simulink model "ComauSMARTS2_CL"  (R2018b)
settings: Solver=ode1  StartTime=0.0  StopTime=tf  FixedStep=T  RelTol=1e-3
values from neighbouring files (symbols this model uses):
  dotq0_ = [0 0 0]    [main.m]
  Kd1 = 1e3    (= 1000)    [main.m]
  Kd2 = 5e2    (= 500)    [main.m]
  Kd3 = 200    [main.m]
  Ki1 = 1e1    (= 10)    [main.m]
  Ki2 = 5e1    (= 50)    [main.m]
  Ki3 = 2    [main.m]
  Kp1 = 1e4    (= 10000)    [main.m]
  Kp2 = 5e3    (= 5000)    [main.m]
  Kp3 = 4e3    (= 4000)    [main.m]
  l1 = 0.65    [main.m]
  l2 = 0.6576    [main.m]
  q0_ = [1.4 0.9 1.1]    [main.m]
  qd_ = [pi/2 pi/4 pi/3]    [main.m]
undefined symbols (not defined in the file or in its folder): gamma
libraries: dspmtrx3 x4, dspinverses x1
settings Model: SimulationMode=accelerator  Creator=gpinc  LastModifiedBy=corrado
settings SFSimCC: SimUseLocalCustomCode=off
settings RTWCC: RTWUseLocalCustomCode=off
settings CodeAppCC: StateflowObjectComments=on

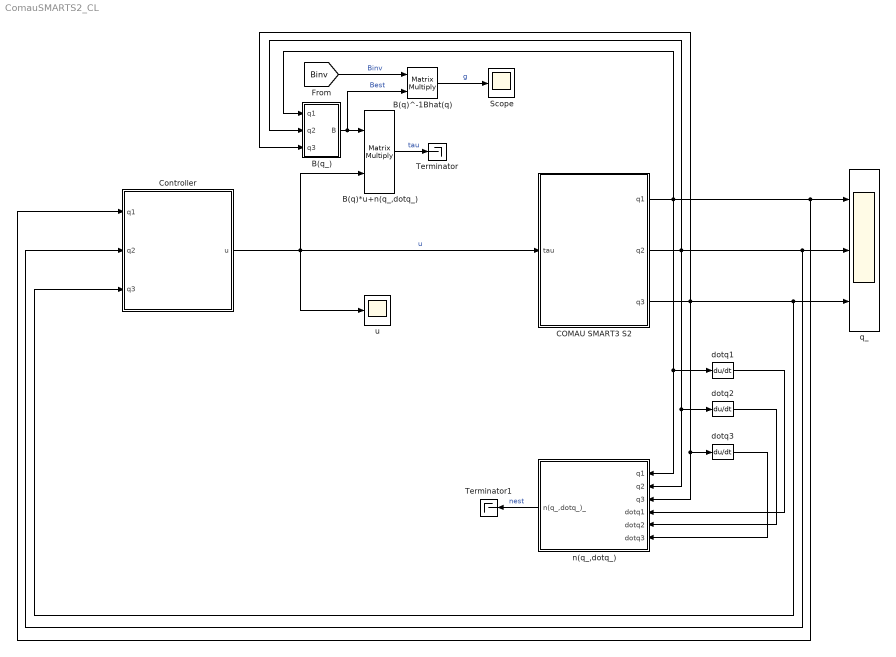
== system ComauSMARTS2_CL ==
  B(q)*u+n(q_,dotq_) : Product  Multiplication=Matrix(*)  RndMeth=Zero
  B(q)^-1Bhat(q) : Product  Multiplication=Matrix(*)  RndMeth=Zero
  B(q_) : Subsystem
  COMAU SMART3 S2 : Subsystem
      mask Display: image(imread('SMARTS2.jpeg'))
  Controller : Subsystem
  Scope : Scope
  Terminator : Terminator
  Terminator1 : Terminator
  dotq1 : Derivative
  dotq2 : Derivative
  dotq3 : Derivative
  n(q_,dotq_) : Subsystem
  q_ : Scope  NumInputPorts=3
  u : Scope
  wires:
  dotq1/1 -> n(q_,dotq_)/4(dotq1)
  B(q_)/1(B) -> B(q)^-1Bhat(q)/2, B(q)*u+n(q_,dotq_)/1  "Best"
  Controller/1(u) -> COMAU SMART3 S2/1(tau), u/1, B(q)*u+n(q_,dotq_)/2  "u"
  COMAU SMART3 S2/2(q2) -> dotq2/1, n(q_,dotq_)/2(q2), B(q_)/2(q2), q_/2, Controller/2(q2)
  dotq3/1 -> n(q_,dotq_)/6(dotq3)
  COMAU SMART3 S2/3(q3) -> dotq3/1, n(q_,dotq_)/3(q3), B(q_)/3(q3), q_/3, Controller/3(q3)
  COMAU SMART3 S2/1(q1) -> dotq1/1, n(q_,dotq_)/1(q1), B(q_)/1(q1), q_/1, Controller/1(q1)
  dotq2/1 -> n(q_,dotq_)/5(dotq2)
  [Binv] -> B(q)^-1Bhat(q)/1  "Binv"
  B(q)^-1Bhat(q)/1 -> Scope/1  "g"
  B(q)*u+n(q_,dotq_)/1 -> Terminator/1  "tau"
  n(q_,dotq_)/1(n(q_,dotq_)_) -> Terminator1/1  "nest"

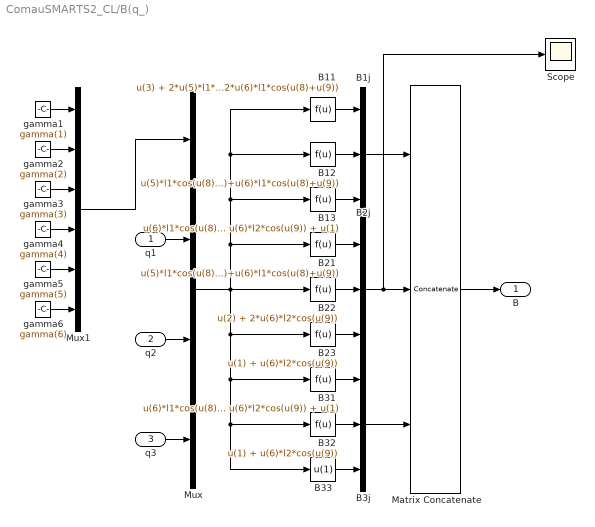
== system ComauSMARTS2_CL/B(q_) ==
  q1 : Inport
  q2 : Inport  Port=2
  q3 : Inport  Port=3
  B11 : Fcn  Expr=u(3) + 2*u(5)*l1*cos(u(8)) + 2*u(6)*l2*cos(u(9)) + 2*u(6)*l1*cos(u(8)+u(9))
  B12 : Fcn  Expr=u(5)*l1*cos(u(8))+u(2)+2*u(6)*l2*cos(u(9))+u(6)*l1*cos(u(8)+u(9))
  B13 : Fcn  Expr=u(6)*l1*cos(u(8)+u(9)) + u(6)*l2*cos(u(9)) + u(1)
  B1j : Concatenate  NumInputs=3
  B21 : Fcn  Expr=u(5)*l1*cos(u(8))+u(2)+2*u(6)*l2*cos(u(9))+u(6)*l1*cos(u(8)+u(9))
  B22 : Fcn  Expr=u(2) + 2*u(6)*l2*cos(u(9))
  B23 : Fcn  Expr=u(1) + u(6)*l2*cos(u(9))
  B2j : Concatenate  NumInputs=3
  B31 : Fcn  Expr=u(6)*l1*cos(u(8)+u(9)) + u(6)*l2*cos(u(9)) + u(1)
  B32 : Fcn  Expr=u(1) + u(6)*l2*cos(u(9))
  B33 : Fcn  Expr=u(1)
  B3j : Concatenate  NumInputs=3
  Matrix Concatenate : Concatenate  NumInputs=3  Mode=Multidimensional array  ConcatenateDimension=2
  Mux : Mux
  Mux1 : Mux  Inputs=6
  Scope : Scope
  gamma1 : Constant  Value=gamma(1)
  gamma2 : Constant  Value=gamma(2)
  gamma3 : Constant  Value=gamma(3)
  gamma4 : Constant  Value=gamma(4)
  gamma5 : Constant  Value=gamma(5)
  gamma6 : Constant  Value=gamma(6)
  B : Outport
  wires:
  B11/1 -> B1j/1
  B33/1 -> B3j/3
  B12/1 -> B1j/2
  B13/1 -> B1j/3
  B22/1 -> B2j/2
  B23/1 -> B2j/3
  B21/1 -> B2j/1
  B31/1 -> B3j/1
  B32/1 -> B3j/2
  Mux/1 -> B22/1, B21/1, B11/1, B12/1, B13/1, B23/1, B31/1, B32/1, B33/1
  Matrix Concatenate/1 -> B/1
  B3j/1 -> Matrix Concatenate/3
  B2j/1 -> Scope/1, Matrix Concatenate/2
  B1j/1 -> Matrix Concatenate/1
  q3/1 -> Mux/4
  q2/1 -> Mux/3
  q1/1 -> Mux/2
  Mux1/1 -> Mux/1
  gamma6/1 -> Mux1/6
  gamma5/1 -> Mux1/5
  gamma4/1 -> Mux1/4
  gamma3/1 -> Mux1/3
  gamma2/1 -> Mux1/2
  gamma1/1 -> Mux1/1

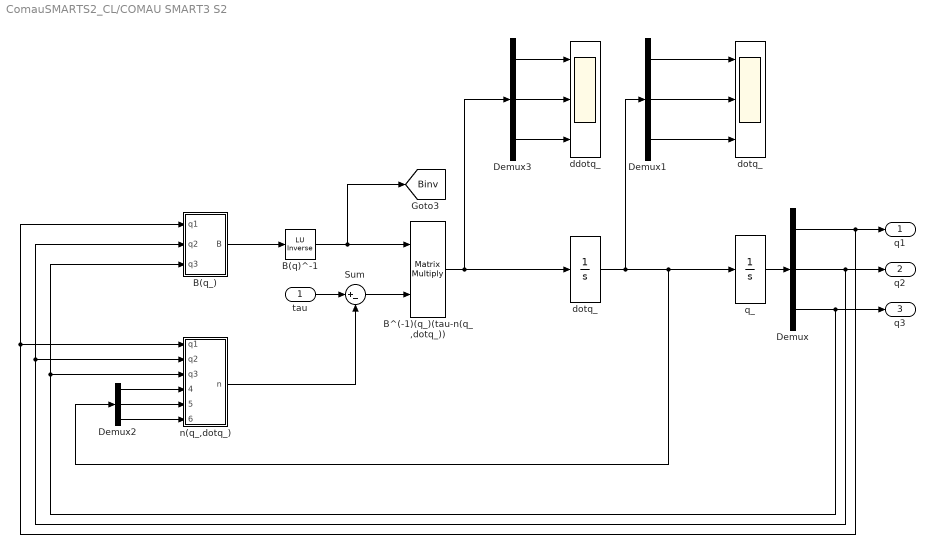
== system ComauSMARTS2_CL/COMAU SMART3 S2 ==
  tau : Inport
  " B(q)^-1" : dspinverses/ LU Inverse
      settings: SourceProductName=DSP System Toolbox
  B(q_) : Subsystem
  B^(-1)(q_)(tau-n(q_,dotq_)) : Product  Multiplication=Matrix(*)  RndMeth=Zero
  Demux{,1..3} (4 alike) : Demux  Outputs=3
  Sum : Sum  Inputs=|+-
  ddotq_ : Scope  NumInputPorts=3
  dotq_ : Integrator  InitialCondition=dotq0_
  "dotq_ " : Scope  NumInputPorts=3
  n(q_,dotq_) : Subsystem
  q_ : Integrator  InitialCondition=q0_
  q1 : Outport
  q2 : Outport  Port=2
  q3 : Outport  Port=3
  tag scope: Binv=global
  wires:
  dotq_/1 -> q_/1, Demux2/1, Demux1/1
  q_/1 -> Demux/1
  B(q_)/1(B) -> " B(q)^-1"/1
  Demux/3 -> q3/1, B(q_)/3(q3), n(q_,dotq_)/3(q3)
  Demux/2 -> q2/1, B(q_)/2(q2), n(q_,dotq_)/2(q2)
  Demux/1 -> q1/1, B(q_)/1(q1), n(q_,dotq_)/1(q1)
  Demux1/3 -> "dotq_ "/3
  Demux1/2 -> "dotq_ "/2
  Demux1/1 -> "dotq_ "/1
  n(q_,dotq_)/1(n) -> Sum/2
  " B(q)^-1"/1 -> [Binv], B^(-1)(q_)(tau-n(q_,dotq_))/1
  Sum/1 -> B^(-1)(q_)(tau-n(q_,dotq_))/2
  Demux3/3 -> ddotq_/3
  Demux3/2 -> ddotq_/2
  tau/1 -> Sum/1
  Demux2/1 -> n(q_,dotq_)/4(dotq1)
  Demux3/1 -> ddotq_/1
  B^(-1)(q_)(tau-n(q_,dotq_))/1 -> Demux3/1, dotq_/1
  Demux2/2 -> n(q_,dotq_)/5(dotq2)
  Demux2/3 -> n(q_,dotq_)/6(dotq3)

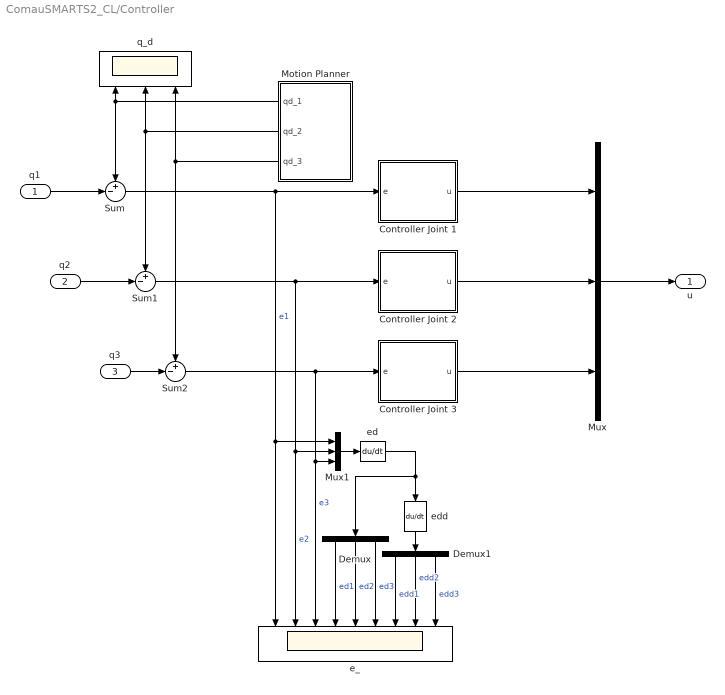
== system ComauSMARTS2_CL/Controller ==
  q1 : Inport
  q2 : Inport  Port=2
  q3 : Inport  Port=3
  Controller Joint 1 : Subsystem
  Controller Joint 2 : Subsystem
  Controller Joint 3 : Subsystem
  Demux : Demux  Outputs=3
  Demux1 : Demux  Outputs=3
  Motion Planner : Subsystem
  Mux : Mux  Inputs=3
  Mux1 : Mux  Inputs=3
  Sum : Sum  Inputs=+-|
  Sum1 : Sum  Inputs=+-|
  Sum2 : Sum  Inputs=+-|
  e_ : Scope  NumInputPorts=9
  ed : Derivative
  edd : Derivative
  q_d : Scope  NumInputPorts=3
  u : Outport
  wires:
  q1/1 -> Sum/2
  q2/1 -> Sum1/2
  q3/1 -> Sum2/2
  Sum/1 -> e_/1, Mux1/1, Controller Joint 1/1(e)  "e1"
  Sum1/1 -> e_/2, Mux1/2, Controller Joint 2/1(e)  "e2"
  Controller Joint 3/1(u) -> Mux/3
  Sum2/1 -> Controller Joint 3/1(e), e_/3, Mux1/3  "e3"
  Mux1/1 -> ed/1
  Demux/1 -> e_/4  "ed1"
  Demux/2 -> e_/5  "ed2"
  Demux/3 -> e_/6  "ed3"
  Demux1/1 -> e_/7  "edd1"
  Demux1/2 -> e_/8  "edd2"
  Demux1/3 -> e_/9  "edd3"
  Controller Joint 2/1(u) -> Mux/2
  Controller Joint 1/1(u) -> Mux/1
  edd/1 -> Demux1/1
  ed/1 -> edd/1, Demux/1
  Mux/1 -> u/1
  Motion Planner/3(qd_3) -> q_d/3, Sum2/1
  Motion Planner/2(qd_2) -> Sum1/1, q_d/2
  Motion Planner/1(qd_1) -> q_d/1, Sum/1

== system ComauSMARTS2_CL/n(q_,dotq_) ==
  q1 : Inport
  q2 : Inport  Port=2
  q3 : Inport  Port=3
  dotq1 : Inport  Port=4
  dotq2 : Inport  Port=5
  dotq3 : Inport  Port=6
  n(q_,dotq_) : Subsystem
  n(q_,dotq_)_ : Outport
  wires:
  q1/1 -> n(q_,dotq_)/1(q1)
  q2/1 -> n(q_,dotq_)/2(q2)
  q3/1 -> n(q_,dotq_)/3(q3)
  n(q_,dotq_)/1(n) -> n(q_,dotq_)_/1
  dotq1/1 -> n(q_,dotq_)/4(dotq1)
  dotq2/1 -> n(q_,dotq_)/5(dotq2)
  dotq3/1 -> n(q_,dotq_)/6(dotq3)

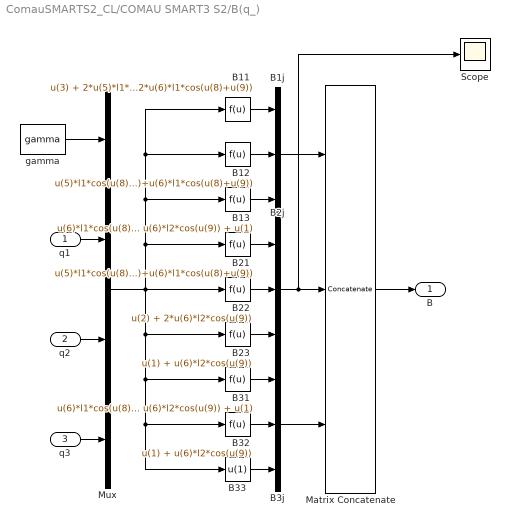
== system ComauSMARTS2_CL/COMAU SMART3 S2/B(q_) ==
  q1 : Inport
  q2 : Inport  Port=2
  q3 : Inport  Port=3
  B11 : Fcn  Expr=u(3) + 2*u(5)*l1*cos(u(8)) + 2*u(6)*l2*cos(u(9)) + 2*u(6)*l1*cos(u(8)+u(9))
  B12 : Fcn  Expr=u(5)*l1*cos(u(8))+u(2)+2*u(6)*l2*cos(u(9))+u(6)*l1*cos(u(8)+u(9))
  B13 : Fcn  Expr=u(6)*l1*cos(u(8)+u(9)) + u(6)*l2*cos(u(9)) + u(1)
  B1j : Concatenate  NumInputs=3
  B21 : Fcn  Expr=u(5)*l1*cos(u(8))+u(2)+2*u(6)*l2*cos(u(9))+u(6)*l1*cos(u(8)+u(9))
  B22 : Fcn  Expr=u(2) + 2*u(6)*l2*cos(u(9))
  B23 : Fcn  Expr=u(1) + u(6)*l2*cos(u(9))
  B2j : Concatenate  NumInputs=3
  B31 : Fcn  Expr=u(6)*l1*cos(u(8)+u(9)) + u(6)*l2*cos(u(9)) + u(1)
  B32 : Fcn  Expr=u(1) + u(6)*l2*cos(u(9))
  B33 : Fcn  Expr=u(1)
  B3j : Concatenate  NumInputs=3
  Matrix Concatenate : Concatenate  NumInputs=3  Mode=Multidimensional array  ConcatenateDimension=2
  Mux : Mux
  Scope : Scope
  gamma : Constant  Value=gamma
  B : Outport
  wires:
  B11/1 -> B1j/1
  B33/1 -> B3j/3
  B12/1 -> B1j/2
  B13/1 -> B1j/3
  B22/1 -> B2j/2
  B23/1 -> B2j/3
  B21/1 -> B2j/1
  B31/1 -> B3j/1
  B32/1 -> B3j/2
  Mux/1 -> B22/1, B21/1, B11/1, B12/1, B13/1, B23/1, B31/1, B32/1, B33/1
  Matrix Concatenate/1 -> B/1
  B3j/1 -> Matrix Concatenate/3
  B2j/1 -> Scope/1, Matrix Concatenate/2
  B1j/1 -> Matrix Concatenate/1
  q3/1 -> Mux/4
  q2/1 -> Mux/3
  q1/1 -> Mux/2
  gamma/1 -> Mux/1

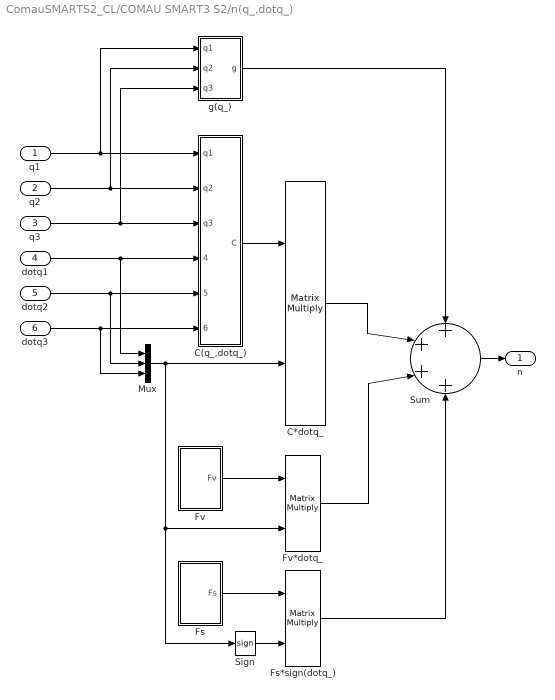
== system ComauSMARTS2_CL/COMAU SMART3 S2/n(q_,dotq_) ==
  q1 : Inport
  q2 : Inport  Port=2
  q3 : Inport  Port=3
  dotq1 : Inport  Port=4
  dotq2 : Inport  Port=5
  dotq3 : Inport  Port=6
  C(q_,dotq_) : Subsystem
  C*dotq_ : Product  Multiplication=Matrix(*)  RndMeth=Zero
  Fs : Subsystem
  Fs*sign(dotq_) : Product  Multiplication=Matrix(*)  RndMeth=Zero
  Fv : Subsystem
  Fv*dotq_ : Product  Multiplication=Matrix(*)  RndMeth=Zero
  Mux : Mux  Inputs=3
  Sign : Signum
  Sum : Sum  Inputs=++++
  g(q_) : Subsystem
  n : Outport
  wires:
  Fv/1(Fv) -> Fv*dotq_/1
  Fs/1(Fs) -> Fs*sign(dotq_)/1
  C(q_,dotq_)/1(C) -> C*dotq_/1
  Sum/1 -> n/1
  Fs*sign(dotq_)/1 -> Sum/4
  C*dotq_/1 -> Sum/2
  g(q_)/1(g) -> Sum/1
  q1/1 -> g(q_)/1(q1), C(q_,dotq_)/1(q1)
  q2/1 -> C(q_,dotq_)/2(q2), g(q_)/2(q2)
  q3/1 -> C(q_,dotq_)/3(q3), g(q_)/3(q3)
  dotq1/1 -> C(q_,dotq_)/4(dotq1), Mux/1
  dotq2/1 -> C(q_,dotq_)/5(dotq2), Mux/2
  dotq3/1 -> C(q_,dotq_)/6(dotq3), Mux/3
  Mux/1 -> C*dotq_/2, Fv*dotq_/2, Sign/1
  Sign/1 -> Fs*sign(dotq_)/2
  Fv*dotq_/1 -> Sum/3

== system ComauSMARTS2_CL/Controller/Controller Joint 1 ==
  e : Inport
  PD : Subsystem
  u : Outport
  wires:
  e/1 -> PD/1(e)
  PD/1(u) -> u/1

== system ComauSMARTS2_CL/Controller/Controller Joint 2 ==
  e : Inport
  PD : Subsystem
  u : Outport
  wires:
  e/1 -> PD/1(e)
  PD/1(u) -> u/1

== system ComauSMARTS2_CL/Controller/Controller Joint 3 ==
  e : Inport
  PD : Subsystem
  u : Outport
  wires:
  PD/1(u) -> u/1
  e/1 -> PD/1(e)

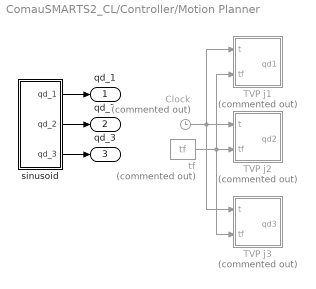
== system ComauSMARTS2_CL/Controller/Motion Planner ==
  " TVP j1" : MATLAB Function  Commented=on  TreatAsAtomicUnit=on
  " TVP j2" : MATLAB Function  Commented=on  TreatAsAtomicUnit=on
  " TVP j3" : MATLAB Function  Commented=on  TreatAsAtomicUnit=on
  Clock : Clock  Commented=on
  sinusoid : Subsystem
  tf : Constant  Commented=on  Value=tf
  qd_1 : Outport
  qd_2 : Outport  Port=2
  qd_3 : Outport  Port=3
  wires:
  Clock/1 -> " TVP j1"/1(t), " TVP j3"/1(t), " TVP j2"/1(t)
  tf/1 -> " TVP j3"/2(tf), " TVP j1"/2(tf), " TVP j2"/2(tf)
  sinusoid/1(qd_1) -> qd_1/1
  sinusoid/2(qd_2) -> qd_2/1
  sinusoid/3(qd_3) -> qd_3/1

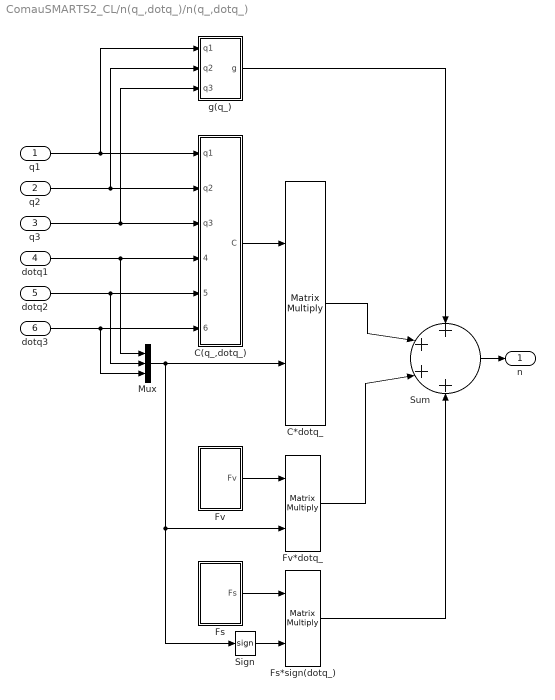
== system ComauSMARTS2_CL/n(q_,dotq_)/n(q_,dotq_) ==
  q1 : Inport
  q2 : Inport  Port=2
  q3 : Inport  Port=3
  dotq1 : Inport  Port=4
  dotq2 : Inport  Port=5
  dotq3 : Inport  Port=6
  C(q_,dotq_) : Subsystem
  C*dotq_ : Product  Multiplication=Matrix(*)  RndMeth=Zero
  Fs : Subsystem
  Fs*sign(dotq_) : Product  Multiplication=Matrix(*)  RndMeth=Zero
  Fv : Subsystem
  Fv*dotq_ : Product  Multiplication=Matrix(*)  RndMeth=Zero
  Mux : Mux  Inputs=3
  Sign : Signum
  Sum : Sum  Inputs=++++
  g(q_) : Subsystem
  n : Outport
  wires:
  Fv/1(Fv) -> Fv*dotq_/1
  Fs/1(Fs) -> Fs*sign(dotq_)/1
  C(q_,dotq_)/1(C) -> C*dotq_/1
  Sum/1 -> n/1
  Fs*sign(dotq_)/1 -> Sum/4
  C*dotq_/1 -> Sum/2
  g(q_)/1(g) -> Sum/1
  q1/1 -> C(q_,dotq_)/1(q1), g(q_)/1(q1)
  q2/1 -> C(q_,dotq_)/2(q2), g(q_)/2(q2)
  q3/1 -> C(q_,dotq_)/3(q3), g(q_)/3(q3)
  Fv*dotq_/1 -> Sum/3
  dotq1/1 -> C(q_,dotq_)/4(dotq1), Mux/1
  dotq2/1 -> C(q_,dotq_)/5(dotq2), Mux/2
  dotq3/1 -> C(q_,dotq_)/6(dotq3), Mux/3
  Mux/1 -> C*dotq_/2, Fv*dotq_/2, Sign/1
  Sign/1 -> Fs*sign(dotq_)/2

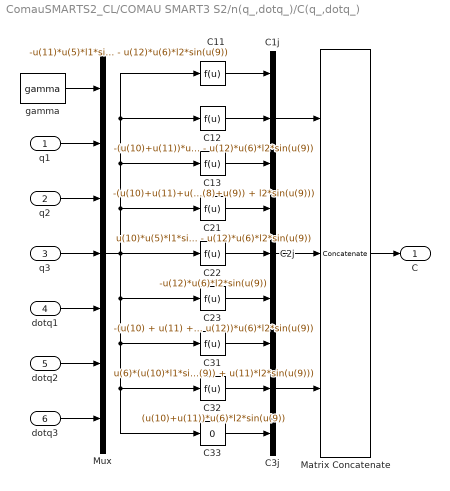
== system ComauSMARTS2_CL/COMAU SMART3 S2/n(q_,dotq_)/C(q_,dotq_) ==
  q1 : Inport
  q2 : Inport  Port=2
  q3 : Inport  Port=3
  dotq1 : Inport  Port=4
  dotq2 : Inport  Port=5
  dotq3 : Inport  Port=6
  C11 : Fcn  Expr=-u(11)*u(5)*l1*sin(u(8)) - (u(11)+u(12))*u(6)*l1*sin(u(8)+u(9)) - u(12)*u(6)*l2*sin(u(9))
  C12 : Fcn  Expr=-(u(10)+u(11))*u(5)*l1*sin(u(8)) - (u(10) + u(11) + u(12))*u(6)*l1*sin(u(8)+u(9)) - u(12)*u(6)*l2*sin(u(9))
  C13 : Fcn  Expr=-(u(10)+u(11)+u(12))*u(6)*(l1*sin(u(8)+u(9)) + l2*sin(u(9)))
  C1j : Concatenate  NumInputs=3
  C21 : Fcn  Expr=u(10)*u(5)*l1*sin(u(8)) + u(10)*u(6)*l1*sin(u(8)+u(9)) - u(12)*u(6)*l2*sin(u(9))
  C22 : Fcn  Expr=-u(12)*u(6)*l2*sin(u(9))
  C23 : Fcn  Expr=-(u(10) + u(11) + u(12))*u(6)*l2*sin(u(9))
  C2j : Concatenate  NumInputs=3
  C31 : Fcn  Expr=u(6)*(u(10)*l1*sin(u(8)+u(9)) + u(10)*l2*sin(u(9)) + u(11)*l2*sin(u(9)))
  C32 : Fcn  Expr=(u(10)+u(11))*u(6)*l2*sin(u(9))
  C33 : Fcn  Expr=0
  C3j : Concatenate  NumInputs=3
  Matrix Concatenate : Concatenate  NumInputs=3  Mode=Multidimensional array  ConcatenateDimension=2
  Mux : Mux  Inputs=7
  gamma : Constant  Value=gamma
  C : Outport
  wires:
  Mux/1 -> C22/1, C11/1, C12/1, C13/1, C21/1, C23/1, C31/1, C33/1, C32/1
  Matrix Concatenate/1 -> C/1
  C13/1 -> C1j/3
  C23/1 -> C2j/3
  C32/1 -> C3j/2
  C3j/1 -> Matrix Concatenate/3
  C22/1 -> C2j/2
  C11/1 -> C1j/1
  C31/1 -> C3j/1
  C1j/1 -> Matrix Concatenate/1
  C2j/1 -> Matrix Concatenate/2
  C21/1 -> C2j/1
  C12/1 -> C1j/2
  C33/1 -> C3j/3
  q1/1 -> Mux/2
  q2/1 -> Mux/3
  q3/1 -> Mux/4
  dotq1/1 -> Mux/5
  dotq2/1 -> Mux/6
  dotq3/1 -> Mux/7
  gamma/1 -> Mux/1

== system ComauSMARTS2_CL/COMAU SMART3 S2/n(q_,dotq_)/Fs ==
  Create Diagonal Matrix : dspmtrx3/Create Diagonal Matrix
      settings: SourceProductName=DSP System Toolbox  SourceProductBaseCode=DS
  Fs11 : Constant  Value=66.3430
  Fs22 : Constant  Value=14.7050
  Fs33 : Constant  Value=8.2911
  Vector Concatenate : Concatenate  NumInputs=3
  Fs : Outport
  wires:
  Fs11/1 -> Vector Concatenate/1
  Fs33/1 -> Vector Concatenate/3
  Fs22/1 -> Vector Concatenate/2
  Create Diagonal Matrix/1 -> Fs/1
  Vector Concatenate/1 -> Create Diagonal Matrix/1

== system ComauSMARTS2_CL/COMAU SMART3 S2/n(q_,dotq_)/Fv ==
  Create Diagonal Matrix : dspmtrx3/Create Diagonal Matrix
      settings: SourceProductName=DSP System Toolbox  SourceProductBaseCode=DS
  Fv11 : Constant  Value=190.4790
  Fv22 : Constant  Value=20.9745
  Fv33 : Constant  Value=4.6565
  Vector Concatenate : Concatenate  NumInputs=3
  Fv : Outport
  wires:
  Create Diagonal Matrix/1 -> Fv/1
  Vector Concatenate/1 -> Create Diagonal Matrix/1
  Fv11/1 -> Vector Concatenate/1
  Fv22/1 -> Vector Concatenate/2
  Fv33/1 -> Vector Concatenate/3

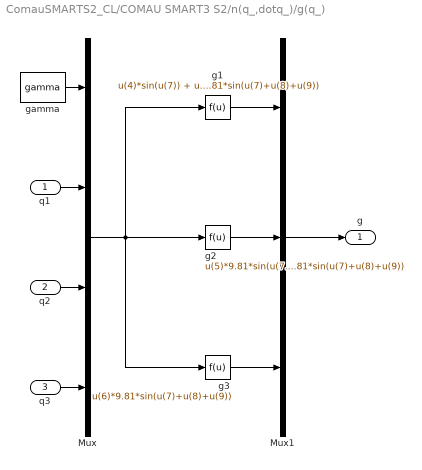
== system ComauSMARTS2_CL/COMAU SMART3 S2/n(q_,dotq_)/g(q_) ==
  q1 : Inport
  q2 : Inport  Port=2
  q3 : Inport  Port=3
  Mux : Mux
  Mux1 : Mux  Inputs=3
  g1 : Fcn  Expr=u(4)*sin(u(7)) + u(5)*9.81*sin(u(7)+u(8)) + u(6)*9.81*sin(u(7)+u(8)+u(9))
  g2 : Fcn  Expr=u(5)*9.81*sin(u(7)+u(8)) + u(6)*9.81*sin(u(7)+u(8)+u(9))
  g3 : Fcn  Expr=u(6)*9.81*sin(u(7)+u(8)+u(9))
  gamma : Constant  Value=gamma
  g : Outport
  wires:
  g1/1 -> Mux1/1
  g2/1 -> Mux1/2
  g3/1 -> Mux1/3
  Mux/1 -> g2/1, g1/1, g3/1
  Mux1/1 -> g/1
  q3/1 -> Mux/4
  q2/1 -> Mux/3
  q1/1 -> Mux/2
  gamma/1 -> Mux/1

== system ComauSMARTS2_CL/Controller/Controller Joint 1/PD ==
  e : Inport
  Integrator : Integrator
  Kd : Gain  Gain=Kd1
  Kd1 : Gain  Gain=Ki1
  Kp : Gain  Gain=Kp1
  Sum2 : Sum  Inputs=+++
  ed : Derivative
  u : Outport
  wires:
  e/1 -> Kp/1, Integrator/1, ed/1
  Sum2/1 -> u/1
  ed/1 -> Kd/1
  Kp/1 -> Sum2/1
  Kd/1 -> Sum2/2
  Integrator/1 -> Kd1/1
  Kd1/1 -> Sum2/3

== system ComauSMARTS2_CL/Controller/Controller Joint 2/PD ==
  e : Inport
  Integrator : Integrator
  Kd : Gain  Gain=Kd2
  Kd1 : Gain  Gain=Ki2
  Kp : Gain  Gain=Kp2
  Sum2 : Sum  Inputs=+++
  ed : Derivative
  u : Outport
  wires:
  e/1 -> Kp/1, Integrator/1, ed/1
  Sum2/1 -> u/1
  ed/1 -> Kd/1
  Kp/1 -> Sum2/1
  Kd/1 -> Sum2/2
  Integrator/1 -> Kd1/1
  Kd1/1 -> Sum2/3

== system ComauSMARTS2_CL/Controller/Controller Joint 3/PD ==
  e : Inport
  Integrator : Integrator
  Kd : Gain  Gain=Kd3
  Kd1 : Gain  Gain=Ki3
  Kp : Gain  Gain=Kp3
  Sum2 : Sum  Inputs=+++
  ed : Derivative
  u : Outport
  wires:
  e/1 -> Kp/1, Integrator/1, ed/1
  Sum2/1 -> u/1
  ed/1 -> Kd/1
  Kp/1 -> Sum2/1
  Kd/1 -> Sum2/2
  Integrator/1 -> Kd1/1
  Kd1/1 -> Sum2/3

== system ComauSMARTS2_CL/Controller/Motion Planner/sinusoid ==
  Constant : Constant  Value=qd_(1)
  Constant1 : Constant  Value=qd_(2)
  Constant2 : Constant  Value=qd_(3)
  qd_1 : Outport
  qd_2 : Outport  Port=2
  qd_3 : Outport  Port=3
  wires:
  Constant1/1 -> qd_2/1
  Constant2/1 -> qd_3/1
  Constant/1 -> qd_1/1

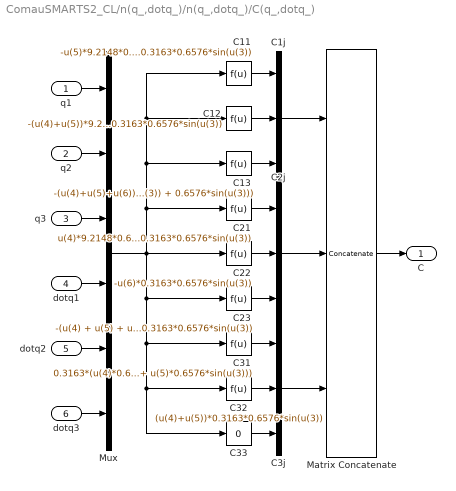
== system ComauSMARTS2_CL/n(q_,dotq_)/n(q_,dotq_)/C(q_,dotq_) ==
  q1 : Inport
  q2 : Inport  Port=2
  q3 : Inport  Port=3
  dotq1 : Inport  Port=4
  dotq2 : Inport  Port=5
  dotq3 : Inport  Port=6
  C11 : Fcn  Expr=-u(5)*9.2148*0.65*sin(u(2)) - (u(5)+u(6))*0.3163*0.65*sin(u(2)+u(3)) - u(6)*0.3163*0.6576*sin(u(3))
  C12 : Fcn  Expr=-(u(4)+u(5))*9.2148*0.65*sin(u(2)) - (u(4) + u(5) + u(6))*0.3163*0.65*sin(u(2)+u(3)) - u(6)*0.3163*0.6576*sin(u(3))
  C13 : Fcn  Expr=-(u(4)+u(5)+u(6))*0.3163*(0.65*sin(u(2)+u(3)) + 0.6576*sin(u(3)))
  C1j : Concatenate  NumInputs=3
  C21 : Fcn  Expr=u(4)*9.2148*0.65*sin(u(2)) + u(4)*0.3163*0.65*sin(u(2)+u(3)) - u(6)*0.3163*0.6576*sin(u(3))
  C22 : Fcn  Expr=-u(6)*0.3163*0.6576*sin(u(3))
  C23 : Fcn  Expr=-(u(4) + u(5) + u(6))*0.3163*0.6576*sin(u(3))
  C2j : Concatenate  NumInputs=3
  C31 : Fcn  Expr=0.3163*(u(4)*0.65*sin(u(2)+u(3)) + u(4)*0.6576*sin(u(3)) + u(5)*0.6576*sin(u(3)))
  C32 : Fcn  Expr=(u(4)+u(5))*0.3163*0.6576*sin(u(3))
  C33 : Fcn  Expr=0
  C3j : Concatenate  NumInputs=3
  Matrix Concatenate : Concatenate  NumInputs=3  Mode=Multidimensional array  ConcatenateDimension=2
  Mux : Mux  Inputs=6
  C : Outport
  wires:
  Mux/1 -> C22/1, C11/1, C12/1, C13/1, C21/1, C23/1, C31/1, C33/1, C32/1
  q1/1 -> Mux/1
  Matrix Concatenate/1 -> C/1
  q2/1 -> Mux/2
  q3/1 -> Mux/3
  dotq1/1 -> Mux/4
  dotq2/1 -> Mux/5
  dotq3/1 -> Mux/6
  C13/1 -> C1j/3
  C23/1 -> C2j/3
  C32/1 -> C3j/2
  C3j/1 -> Matrix Concatenate/3
  C22/1 -> C2j/2
  C11/1 -> C1j/1
  C31/1 -> C3j/1
  C1j/1 -> Matrix Concatenate/1
  C2j/1 -> Matrix Concatenate/2
  C21/1 -> C2j/1
  C12/1 -> C1j/2
  C33/1 -> C3j/3

== system ComauSMARTS2_CL/n(q_,dotq_)/n(q_,dotq_)/Fs ==
  Create Diagonal Matrix : dspmtrx3/Create Diagonal Matrix
      settings: SourceProductName=DSP System Toolbox  SourceProductBaseCode=DS
  Fs11 : Constant  Value=66.3430
  Fs22 : Constant  Value=14.7050
  Fs33 : Constant  Value=8.2911
  Vector Concatenate : Concatenate  NumInputs=3
  Fs : Outport
  wires:
  Fs11/1 -> Vector Concatenate/1
  Fs33/1 -> Vector Concatenate/3
  Fs22/1 -> Vector Concatenate/2
  Create Diagonal Matrix/1 -> Fs/1
  Vector Concatenate/1 -> Create Diagonal Matrix/1

== system ComauSMARTS2_CL/n(q_,dotq_)/n(q_,dotq_)/Fv ==
  Create Diagonal Matrix : dspmtrx3/Create Diagonal Matrix
      settings: SourceProductName=DSP System Toolbox  SourceProductBaseCode=DS
  Fv11 : Constant  Value=190.4790
  Fv22 : Constant  Value=20.9745
  Fv33 : Constant  Value=4.6565
  Vector Concatenate : Concatenate  NumInputs=3
  Fv : Outport
  wires:
  Fv11/1 -> Vector Concatenate/1
  Fv33/1 -> Vector Concatenate/3
  Fv22/1 -> Vector Concatenate/2
  Create Diagonal Matrix/1 -> Fv/1
  Vector Concatenate/1 -> Create Diagonal Matrix/1

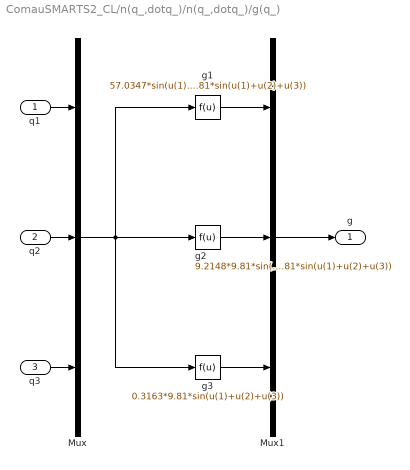
== system ComauSMARTS2_CL/n(q_,dotq_)/n(q_,dotq_)/g(q_) ==
  q1 : Inport
  q2 : Inport  Port=2
  q3 : Inport  Port=3
  Mux : Mux  Inputs=3
  Mux1 : Mux  Inputs=3
  g1 : Fcn  Expr=57.0347*sin(u(1)) + 9.2148*9.81*sin(u(1)+u(2)) + 0.3163*9.81*sin(u(1)+u(2)+u(3))
  g2 : Fcn  Expr=9.2148*9.81*sin(u(1)+u(2)) + 0.3163*9.81*sin(u(1)+u(2)+u(3))
  g3 : Fcn  Expr=0.3163*9.81*sin(u(1)+u(2)+u(3))
  g : Outport
  wires:
  g1/1 -> Mux1/1
  g2/1 -> Mux1/2
  g3/1 -> Mux1/3
  Mux/1 -> g2/1, g1/1, g3/1
  q1/1 -> Mux/1
  Mux1/1 -> g/1
  q2/1 -> Mux/2
  q3/1 -> Mux/3

== matlab function ComauSMARTS2_CL/Controller/Motion Planner/ TVP j1 ==
  data: t input; qd1 output; tf input
function qd1 = fcn(t,tf)

qd1 =0;

if t <=2*tf/3
    
    qi = 0;
    qf = pi/8;
    
    ti = 0;
    t_f = 2*tf/3;
    
    dqv = 1.1*abs(qf-qi)/(t_f-ti);
    ddqv = (dqv^2)/(qi-qf+dqv*(t_f-ti));
    ta = (qi-qf+dqv*(t_f-ti))/(dqv);
    
    
    % TVP  function
    
    if t>= ti && t<= ti+ta
        qd1 = qi+0.5*ddqv*(t-ti)^2;
    elseif t> ti+ta && t<= t_f-ta
        qd1 = qi+ddqv*ta*(t-ti-ta/2);
    elseif t<= t_f && t> t_f-ta
        qd1 = qf-0.5*ddqv*(t_f-t)^2;
    end
    
else
    
    qi = pi/8;
    qf = 0;
    
    ti = 2*tf/3;
    t_f = tf;
    
    dqv = -1.1*abs(qf-qi)/(t_f-ti);
    ddqv = (dqv^2)/(qi-qf+dqv*(t_f-ti));
    ta = (qi-qf+dqv*(t_f-ti))/(dqv);
    
    
    % TVP  function
    
    if t>= ti && t<= ti+ta
        qd1 = qi+0.5*ddqv*(t-ti)^2;
    elseif t> ti+ta && t<= t_f-ta
        qd1 = qi+ddqv*ta*(t-ti-ta/2);
    elseif t<= t_f && t> t_f-ta
        qd1 = qf-0.5*ddqv*(t_f-t)^2;
    end
    
end

== matlab function ComauSMARTS2_CL/Controller/Motion Planner/ TVP j2 ==
  data: t input; qd2 output; tf input
function qd2 = fcn(t,tf)


qd2 =0;

if t <=2*tf/3
    
    qi = 0;
    qf = pi/8;
    
    ti = 0;
    t_f = 2*tf/3;
    
    dqv = 1.1*abs(qf-qi)/(t_f-ti);
    ddqv = (dqv^2)/(qi-qf+dqv*(t_f-ti));
    ta = (qi-qf+dqv*(t_f-ti))/(dqv);
    
    
    % TVP  function
    
    if t>= ti && t<= ti+ta
        qd2 = qi+0.5*ddqv*(t-ti)^2;
    elseif t> ti+ta && t<= t_f-ta
        qd2 = qi+ddqv*ta*(t-ti-ta/2);
    elseif t<= t_f && t> t_f-ta
        qd2 = qf-0.5*ddqv*(t_f-t)^2;
    end
    
else
    
    qi = pi/8;
    qf = 0;
    
    ti = 2*tf/3;
    t_f = tf;
    
    dqv = -1.1*abs(qf-qi)/(t_f-ti);
    ddqv = (dqv^2)/(qi-qf+dqv*(t_f-ti));
    ta = (qi-qf+dqv*(t_f-ti))/(dqv);
    
    
    % TVP  function
    
    if t>= ti && t<= ti+ta
        qd2 = qi+0.5*ddqv*(t-ti)^2;
    elseif t> ti+ta && t<= t_f-ta
        qd2 = qi+ddqv*ta*(t-ti-ta/2);
    elseif t<= t_f && t> t_f-ta
        qd2 = qf-0.5*ddqv*(t_f-t)^2;
    end
    
end

== matlab function ComauSMARTS2_CL/Controller/Motion Planner/ TVP j3 ==
  data: t input; qd3 output; tf input
function qd3 = fcn(t,tf)

qd3 =0;

if t <=tf/2
    
    qi = pi/2;
    qf = pi/4;
    
    ti = 0;
    t_f = tf/2;
    
    dqv = -1.1*abs(qf-qi)/(t_f-ti);
    ddqv = (dqv^2)/(qi-qf+dqv*(t_f-ti));
    ta = (qi-qf+dqv*(t_f-ti))/(dqv);
    
    
    % TVP  function
    
    if t>= ti && t<= ti+ta
        qd3 = qi+0.5*ddqv*(t-ti)^2;
    elseif t> ti+ta && t<= t_f-ta
        qd3 = qi+ddqv*ta*(t-ti-ta/2);
    elseif t<= t_f && t> t_f-ta
        qd3 = qf-0.5*ddqv*(t_f-t)^2;
    end
    
else
    
    qi = pi/4;
    qf = pi/2;
    
    ti = tf/2;
    t_f = tf;
    
    dqv = 1.1*abs(qf-qi)/(t_f-ti);
    ddqv = (dqv^2)/(qi-qf+dqv*(t_f-ti));
    ta = (qi-qf+dqv*(t_f-ti))/(dqv);
    
    
    % TVP  function
    
    if t>= ti && t<= ti+ta
        qd3 = qi+0.5*ddqv*(t-ti)^2;
    elseif t> ti+ta && t<= t_f-ta
        qd3 = qi+ddqv*ta*(t-ti-ta/2);
    elseif t<= t_f && t> t_f-ta
        qd3 = qf-0.5*ddqv*(t_f-t)^2;
    end
    
end
